simulink model "PlantIdentificationMPC"  (R2025b)
settings: Solver=ode14x  StartTime=0.0  StopTime=4 * seqLen * Ts_ctrl  FixedStep=Ts_local  RelTol=1e-3
model workspace (MAT data in the model file):
  A = 0.03
  Tg = 20
  Tp = 10
  seqLen = 511
undefined symbols (not defined in the file or in its folder): Ts_ctrl
settings Model: DataDictionary=ctrlSys.sldd  Creator=LYG  LastModifiedBy=mercer

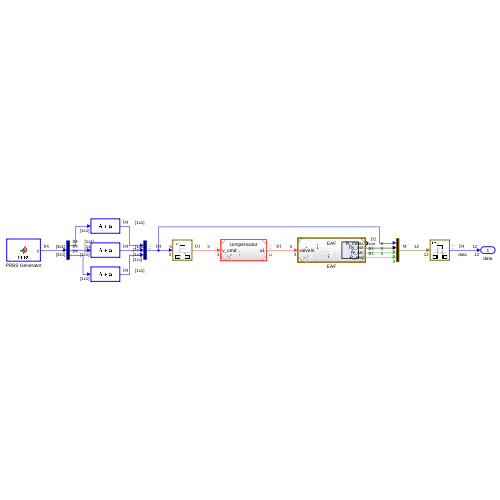
[thumbnail: Simulink's stored preview of the top-level diagram]
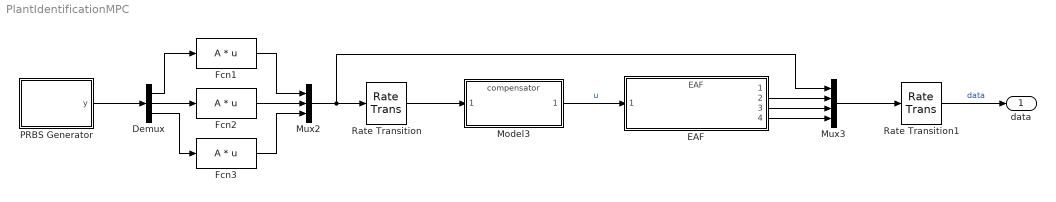
== system PlantIdentificationMPC ==
  Demux : Demux  Outputs=3
  EAF : ModelReference  ModelNameDialog=EAF.slx  SimulationMode=Normal  ModelReferenceVersion=1.82
  Fcn1 : Fcn  Expr=A * u
  Fcn2 : Fcn  Expr=A * u
  Fcn3 : Fcn  Expr=A * u
  Model3 : ModelReference  ModelNameDialog=compensator.slx  SimulationMode=Normal  ModelReferenceVersion=1.22
  Mux2 : Mux  Inputs=3
  Mux3 : Mux
  PRBS Generator : MATLAB Function  TreatAsAtomicUnit=on  SystemSampleTime=Ts_ctrl
  Rate Transition : RateTransition  OutPortSampleTime=Ts_local
  Rate Transition1 : RateTransition  OutPortSampleTime=Ts_ctrl
  data : Outport
  wires:
  Demux/1 -> Fcn1/1
  Demux/2 -> Fcn2/1
  Demux/3 -> Fcn3/1
  Fcn1/1 -> Mux2/1
  Fcn2/1 -> Mux2/2
  Fcn3/1 -> Mux2/3
  Mux3/1 -> Rate Transition1/1
  Rate Transition/1 -> Model3/1
  Model3/1 -> EAF/1  "u"
  PRBS Generator/1(y) -> Demux/1
  Mux2/1 -> Mux3/1, Rate Transition/1
  EAF/2 -> Mux3/2
  Rate Transition1/1 -> data/1  "data"
  EAF/3 -> Mux3/3
  EAF/4 -> Mux3/4

== matlab function PlantIdentificationMPC/PRBS Generator ==
  data: y output; seqLen parameter size=[1 1]; Tp parameter size=[1 1]; Tg parameter
function y = PRBS(seqLen, Tp, Tg)
% Codegen-friendly PRBS pulse train using LFSRs (max-length).
% Output levels: {-1, 0, +1}.
% Each pulse width is Tp samples, followed by a zero gap of Tg samples.
% Output is a 3x1 vector of independent PRBS signals.

persistent lfsr m phaseCnt isPulse pulseVal

if isempty(lfsr)
    % Choose LFSR order so period >= seqLen
    m = max(2, ceil(log2(double(seqLen) + 1)));
    if m > 16
        m = 16; % limit to supported taps below
    end
    lfsr = uint32([1 7 3]); % non-zero seeds for 3 independent sequences
    lfsr = bitand(lfsr, bitshift(uint32(1), m) - 1);
    lfsr(lfsr == 0) = uint32(1);
    phaseCnt = uint32([0 0 0]);
    isPulse = false(1, 3);
    pulseVal = [0 0 0];
end

tp = uint32(max(1, Tp));
tg = uint32(max(1, Tg));
y = zeros(3, 1);

% Per channel state machine:
% Pulse phase -> output +/-1 for Tp samples
% Gap phase   -> output 0 for Tg samples
for i = 1:3
    if phaseCnt(i) == 0
        if ~isPulse(i)
            % Start a new pulse: advance PRBS and choose pulse sign.
            fb = lfsr_feedback(lfsr(i), m, i);
            lfsr(i) = bitshift(lfsr(i), 1);
            lfsr(i) = bitset(lfsr(i), 1, fb);
            lfsr(i) = bitand(lfsr(i), bitshift(uint32(1), m) - 1);
            pulseVal(i) = 2 * double(bitget(lfsr(i), 1)) - 1; % {-1,+1}
            isPulse(i) = true;
            phaseCnt(i) = tp;
        else
            % Pulse finished: enforce zero gap.
            isPulse(i) = false;
            phaseCnt(i) = tg;
            y(i) = 0;
            phaseCnt(i) = phaseCnt(i) - 1;
            continue
        end
    end

    if isPulse(i)
        y(i) = pulseVal(i);
    else
        y(i) = 0;
    end
    phaseCnt(i) = phaseCnt(i) - 1;
end

end

function fb = lfsr_feedback(s, m, chan)
% Max-length taps for m = 2..16 (Fibonacci form).
% For m = 9, use three different primitive polynomials per channel.
switch m
    case 2
        fb = bitxor(bitget(s,2), bitget(s,1));
    case 3
        fb = bitxor(bitget(s,3), bitget(s,2));
    case 4
        fb = bitxor(bitget(s,4), bitget(s,3));
    case 5
        fb = bitxor(bitget(s,5), bitget(s,3));
    case 6
        fb = bitxor(bitget(s,6), bitget(s,5));
    case 7
        fb = bitxor(bitget(s,7), bitget(s,6));
    case 8
        fb = bitxor(bitxor(bitget(s,8), bitget(s,6)), bitxor(bitget(s,5), bitget(s,4)));
    case 9
        switch chan
            case 1
                % x^9 + x^5 + 1
                fb = bitxor(bitget(s,9), bitget(s,5));
            case 2
                % x^9 + x^4 + 1
                fb = bitxor(bitget(s,9), bitget(s,4));
            otherwise
                % x^9 + x^6 + x^5 + x^2 + 1
                fb = bitxor(bitxor(bitget(s,9), bitget(s,6)), ...
                    bitxor(bitget(s,5), bitget(s,2)));
        end
    case 10
        fb = bitxor(bitget(s,10), bitget(s,7));
    case 11
        fb = bitxor(bitget(s,11), bitget(s,9));
    case 12
        fb = bitxor(bitxor(bitget(s,12), bitget(s,6)), bitxor(bitget(s,4), bitget(s,1)));
    case 13
        fb = bitxor(bitxor(bitget(s,13), bitget(s,4)), bitxor(bitget(s,3), bitget(s,1)));
    case 14
        fb = bitxor(bitxor(bitget(s,14), bitget(s,5)), bitxor(bitget(s,3), bitget(s,1)));
    case 15
        fb = bitxor(bitget(s,15), bitget(s,14));
    otherwise % 16
        fb = bitxor(bitxor(bitget(s,16), bitget(s,15)), bitxor(bitget(s,13), bitget(s,4)));
end
end
